simulink model "LinearTopTest_discrete"  (R2019a)
settings: Solver=VariableStepAuto  StartTime=0.0  StopTime=10  MaxStep=h  RelTol=1e-3
values from neighbouring files (symbols this model uses):
  Parameters = CoenParams(X)    [EstimatedParams.m]    (also in LQR.m = EstimatedParams(); LSQnonLinfunc.m; TestModel.m = CoenParams(X0); testingLQRDisturbance.m = EstimatedParams())
undefined symbols (not defined in the file or in its folder): DiscIntNeverNeededParam
settings Model: Creator=BozeMannen  LastModifiedBy=coeng
settings DataIOCC: ReturnWorkspaceOutputs=off
settings DebuggingCC: PregeneratedLibrarySubsystemCodeDiagnostic=none  ArithmeticOperatorsInVariantConditions=warning
settings SFSimCC: SimUseLocalCustomCode=off
settings RTWCC: RTWUseLocalCustomCode=off

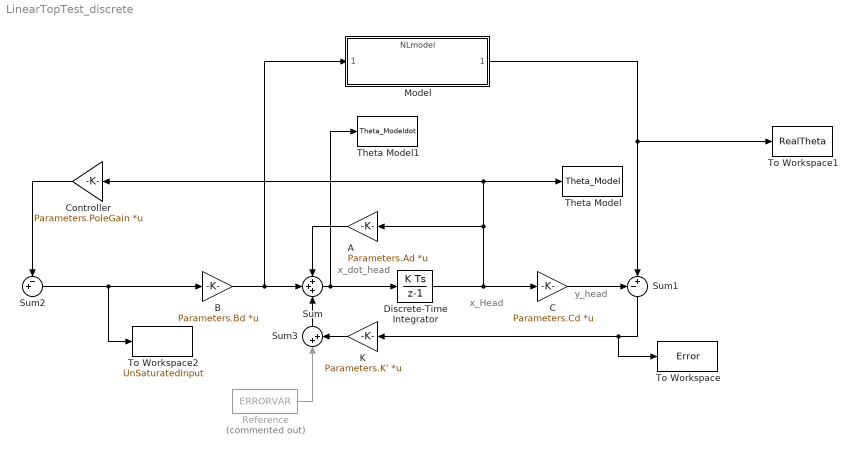
== system LinearTopTest_discrete ==
  note: y_head
  note: x_Head
  note: x_dot_head
  A : Gain  Gain=Parameters.Ad  Multiplication=Matrix(K*u)
  B : Gain  Gain=Parameters.Bd  Multiplication=Matrix(K*u)
  C : Gain  Gain=Parameters.Cd  Multiplication=Matrix(K*u)
  Controller : Gain  Gain=Parameters.PoleGain  Multiplication=Matrix(K*u)
  Discrete-Time Integrator : DiscreteIntegrator  InitialCondition=firstLocation'  SampleTime=-1  ICPrevOutput=DiscIntNeverNeededParam  ICPrevScaledInput=DiscIntNeverNeededParam
  K : Gain  Gain=Parameters.K'  Multiplication=Matrix(K*u)
  Model : ModelReference  ModelNameDialog=NLmodel  SimulationMode=Normal  ModelReferenceVersion=1.67
  "Reference " : FromWorkspace  Commented=on  VariableName=ERRORVAR  SampleTime=0
  Sum : Sum  Inputs=+++
  Sum1 : Sum  Inputs=-+|
  Sum2 : Sum  Inputs=-+|
  Sum3 : Sum  Inputs=|++
  Theta Model : ToWorkspace  VariableName=Theta_Model  SaveFormat=Timeseries  SampleTime=-1
  Theta Model1 : ToWorkspace  VariableName=Theta_Modeldot  SaveFormat=Timeseries  SampleTime=-1
  To Workspace : ToWorkspace  VariableName=Error  SaveFormat=Timeseries  SampleTime=-1
  To Workspace1 : ToWorkspace  VariableName=RealTheta  SaveFormat=Timeseries  SampleTime=-1
  To Workspace2 : ToWorkspace  VariableName=UnSaturatedInput  SaveFormat=Timeseries  SampleTime=-1
  wires:
  "Reference "/1 -> Sum3/1
  K/1 -> Sum3/2
  Sum/1 -> Discrete-Time Integrator/1, Theta Model1/1
  Model/1 -> To Workspace1/1, Sum1/2
  Controller/1 -> Sum2/1
  B/1 -> Model/1, Sum/2
  Discrete-Time Integrator/1 -> C/1, A/1, Controller/1, Theta Model/1
  A/1 -> Sum/1
  C/1 -> Sum1/1
  Sum1/1 -> K/1, To Workspace/1
  Sum2/1 -> B/1, To Workspace2/1
  Sum3/1 -> Sum/3
